simulink model "Lab2_static"  (R2022b)
settings: Solver=VariableStepAuto  StartTime=0.0  StopTime=t  MaxStep=0.01  RelTol=1e-3
undefined symbols (not defined in the file): gamma, lambda, theta, x_0
settings Model: Creator=DuPont  LastModifiedBy=DuPont

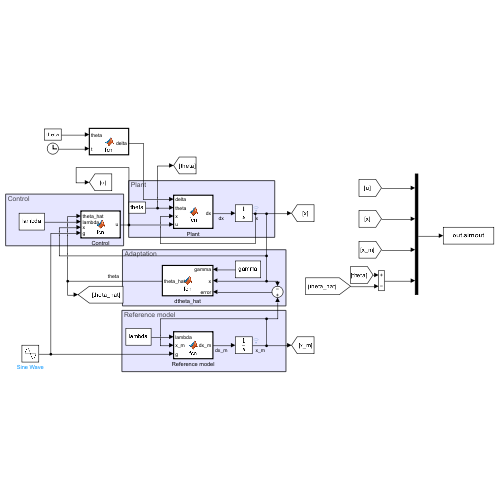
[thumbnail: Simulink's stored preview of the top-level diagram]
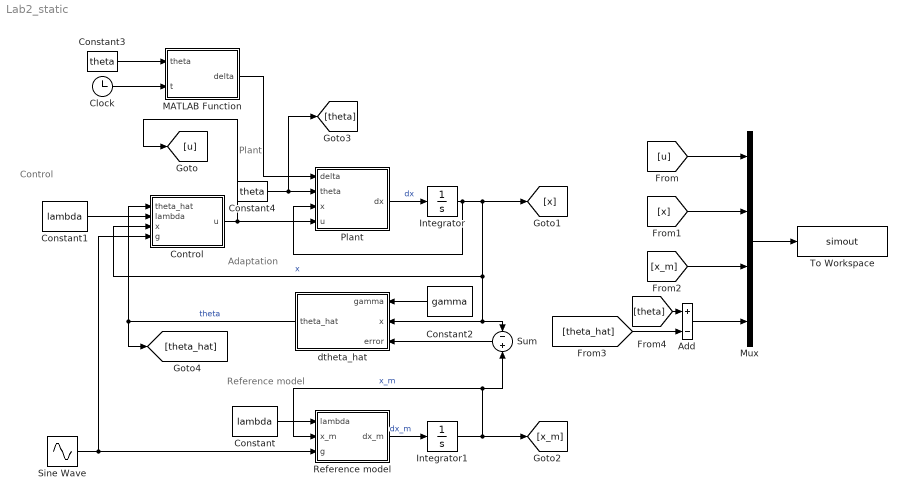
== system Lab2_static ==
  note: Reference model
  note: Adaptation
  note: Control
  note: Plant
  Add : Sum  Inputs=+-
  Clock : Clock
  Constant : Constant  Value=lambda
  Constant1 : Constant  Value=lambda
  Constant2 : Constant  Value=gamma
  Constant3 : Constant  Value=theta
  Constant4 : Constant  Value=theta
  Control : MATLAB Function  TreatAsAtomicUnit=on
  Integrator : Integrator  InitialCondition=x_0
  Integrator1 : Integrator
  MATLAB Function : MATLAB Function  TreatAsAtomicUnit=on
  Mux : Mux
  Plant : MATLAB Function  TreatAsAtomicUnit=on
  Reference model : MATLAB Function  TreatAsAtomicUnit=on
  Sine Wave : Sin  Bias=2  Frequency=8  SampleTime=0
  Sum : Sum  Inputs=-|+
  To Workspace : ToWorkspace  VariableName=simout  SaveFormat=Structure With Time  SampleTime=-1
  dtheta_hat : MATLAB Function  TreatAsAtomicUnit=on
  wires:
  Sine Wave/1 -> Reference model/3(g), Control/4(g)
  Control/1(u) -> [u], Plant/4(u)
  Plant/1(dx) -> Integrator/1  "dx"
  Integrator/1 -> Plant/3(x), Control/3(x), dtheta_hat/2(x), Sum/1, [x]  "x"
  Reference model/1(dx_m) -> Integrator1/1  "dx_m"
  Integrator1/1 -> [x_m], Sum/2, Reference model/2(x_m)  "x_m"
  Constant/1 -> Reference model/1(lambda)
  Constant1/1 -> Control/2(lambda)
  Sum/1 -> dtheta_hat/3(error)
  Constant2/1 -> dtheta_hat/1(gamma)
  dtheta_hat/1(theta_hat) -> [theta_hat], Control/1(theta_hat)  "theta"
  [u] -> Mux/1
  [x] -> Mux/2
  [x_m] -> Mux/3
  [theta_hat] -> Add/2
  [theta] -> Add/1
  Add/1 -> Mux/4
  Mux/1 -> To Workspace/1
  Constant4/1 -> [theta], Plant/2(theta)
  Constant3/1 -> MATLAB Function/1(theta)
  Clock/1 -> MATLAB Function/2(t)
  MATLAB Function/1(delta) -> Plant/1(delta)

== matlab function Lab2_static/Plant ==
  data: delta input; dx output; theta input; x input; u input
function dx = fcn(delta, theta, x , u)

dx = theta*x + u;

== matlab function Lab2_static/Control ==
  data: u output; theta_hat input; lambda input; x input; g input
function u = fcn(theta_hat, lambda, x, g)

u = -theta_hat*x - lambda*x + lambda*g;

== matlab function Lab2_static/Reference model ==
  data: dx_m output; lambda input; x_m input; g input
function dx_m = fcn(lambda, x_m, g)

dx_m = -lambda*x_m + lambda*g;

== matlab function Lab2_static/dtheta_hat ==
  data: theta_hat output; gamma input; x input; error input
function theta_hat  = fcn(gamma, x, error)

theta_hat = -gamma * x * error;

== matlab function Lab2_static/MATLAB Function ==
  data: theta input; delta output; t input
function delta = fcn(theta, t)

delta = (1+t)^(-1/8)*(1-theta*(1+t)^(-1/4)-3/8*(1+t)^(-5/4));
